simulink model "Y_Model_20_Loads"  (R2018b)
settings: Solver=VariableStepAuto  StartTime=0.0  StopTime=sim_t  RelTol=1e-3
values from neighbouring files (symbols this model uses):
  dt = 5e-5    (= 5e-05)    [Y_multi_sim_loads.m]
  L = ones(num_sims, num_loads) * L_max    [Y_multi_sim_loads.m]
  P = rand(num_sims, num_loads) * (P_max - P_min) + P_min    [Y_multi_sim_loads.m]
  R = ones(num_sims, num_loads) * R_max    [Y_multi_sim_loads.m]
libraries: powerlib x270, powerlib_meascontrol x56
(part 4 of 4)

== system Y_Model_20_Loads/PMU 7 ==
  "PMU (PLL-Based, Positive-Sequence)1" : powerlib_meascontrol/Measurements/PMU (PLL-Based, Positive-Sequence)  nominalFrequency=50  samplingRate=64  reportingFactor=64
      settings: SourceProductName=Simscape Electrical  SourceProductBaseCode=PS
  "PMU (PLL-Based, Positive-Sequence)2" : powerlib_meascontrol/Measurements/PMU (PLL-Based, Positive-Sequence)  nominalFrequency=50  samplingRate=64  reportingFactor=64
      settings: SourceProductName=Simscape Electrical  SourceProductBaseCode=PS
  Three-Phase V-I Measurement1 : powerlib/Measurements/Three-Phase V-I Measurement  VoltageMeasurement=phase-to-ground  SetLabelV=off  LabelV=Vabc  Vpu=off  VpuLL=off  CurrentMeasurement=no  SetLabelI=off  LabelI=Iabc  Ipu=off  Pbase=100e6  Vbase=500e3  OutputType=Complex  PhasorSimulation=off  PSBequivalent=0
      settings: SourceProductName=Simscape Electrical
  Three-Phase V-I Measurement25 : powerlib/Measurements/Three-Phase V-I Measurement  VoltageMeasurement=no  SetLabelV=off  LabelV=Vabc  Vpu=off  VpuLL=off  CurrentMeasurement=yes  SetLabelI=off  LabelI=Iabc  Ipu=off  Pbase=100e6  Vbase=500e3  OutputType=Complex  PhasorSimulation=off  PSBequivalent=0
      settings: SourceProductName=Simscape Electrical
  To Workspace1 : ToWorkspace  VariableName=i_mag7  SampleTime=-1
  To Workspace2 : ToWorkspace  VariableName=i_ang7  SampleTime=-1
  To Workspace3 : ToWorkspace  VariableName=v_mag7  SampleTime=-1
  To Workspace4 : ToWorkspace  VariableName=v_ang7  SampleTime=-1
  To Workspace5 : ToWorkspace  VariableName=v_freq7  SampleTime=-1
  To Workspace6 : ToWorkspace  VariableName=i_freq7  SampleTime=-1
  Connection Port : PMIOPort  Tag=PMCPort  Side=Left
  Connection Port1 : PMIOPort  Tag=PMCPort  Port=2  Side=Left
  Connection Port2 : PMIOPort  Tag=PMCPort  Port=3  Side=Left
  Connection Port3 : PMIOPort  Tag=PMCPort  Port=4  Side=Right
  Connection Port4 : PMIOPort  Tag=PMCPort  Port=5  Side=Right
  Connection Port5 : PMIOPort  Tag=PMCPort  Port=6  Side=Right
  wires:
  "PMU (PLL-Based, Positive-Sequence)1"/3 -> To Workspace5/1
  "PMU (PLL-Based, Positive-Sequence)1"/2 -> To Workspace4/1
  "PMU (PLL-Based, Positive-Sequence)1"/1 -> To Workspace3/1
  "PMU (PLL-Based, Positive-Sequence)2"/3 -> To Workspace6/1
  "PMU (PLL-Based, Positive-Sequence)2"/1 -> To Workspace1/1
  "PMU (PLL-Based, Positive-Sequence)2"/2 -> To Workspace2/1
  Three-Phase V-I Measurement25/1 -> "PMU (PLL-Based, Positive-Sequence)2"/1
  Three-Phase V-I Measurement1/1 -> "PMU (PLL-Based, Positive-Sequence)1"/1
  connections:
  Three-Phase V-I Measurement25/LConn1 -- Connection Port/RConn1 -- Three-Phase V-I Measurement1/LConn1
  Connection Port1/RConn1 -- Three-Phase V-I Measurement1/LConn2 -- Three-Phase V-I Measurement25/LConn2
  Connection Port2/RConn1 -- Three-Phase V-I Measurement25/LConn3 -- Three-Phase V-I Measurement1/LConn3
  Connection Port3/RConn1 -- Three-Phase V-I Measurement25/RConn1
  Three-Phase V-I Measurement25/RConn2 -- Connection Port4/RConn1
  Three-Phase V-I Measurement25/RConn3 -- Connection Port5/RConn1

== system Y_Model_20_Loads/PMU 8 ==
  "PMU (PLL-Based, Positive-Sequence)1" : powerlib_meascontrol/Measurements/PMU (PLL-Based, Positive-Sequence)  nominalFrequency=50  samplingRate=64  reportingFactor=64
      settings: SourceProductName=Simscape Electrical  SourceProductBaseCode=PS
  "PMU (PLL-Based, Positive-Sequence)2" : powerlib_meascontrol/Measurements/PMU (PLL-Based, Positive-Sequence)  nominalFrequency=50  samplingRate=64  reportingFactor=64
      settings: SourceProductName=Simscape Electrical  SourceProductBaseCode=PS
  Three-Phase V-I Measurement1 : powerlib/Measurements/Three-Phase V-I Measurement  VoltageMeasurement=phase-to-ground  SetLabelV=off  LabelV=Vabc  Vpu=off  VpuLL=off  CurrentMeasurement=no  SetLabelI=off  LabelI=Iabc  Ipu=off  Pbase=100e6  Vbase=500e3  OutputType=Complex  PhasorSimulation=off  PSBequivalent=0
      settings: SourceProductName=Simscape Electrical
  Three-Phase V-I Measurement25 : powerlib/Measurements/Three-Phase V-I Measurement  VoltageMeasurement=no  SetLabelV=off  LabelV=Vabc  Vpu=off  VpuLL=off  CurrentMeasurement=yes  SetLabelI=off  LabelI=Iabc  Ipu=off  Pbase=100e6  Vbase=500e3  OutputType=Complex  PhasorSimulation=off  PSBequivalent=0
      settings: SourceProductName=Simscape Electrical
  To Workspace1 : ToWorkspace  VariableName=i_mag8  SampleTime=-1
  To Workspace2 : ToWorkspace  VariableName=i_ang8  SampleTime=-1
  To Workspace3 : ToWorkspace  VariableName=v_mag8  SampleTime=-1
  To Workspace4 : ToWorkspace  VariableName=v_ang8  SampleTime=-1
  To Workspace5 : ToWorkspace  VariableName=v_freq8  SampleTime=-1
  To Workspace6 : ToWorkspace  VariableName=i_freq8  SampleTime=-1
  Connection Port : PMIOPort  Tag=PMCPort  Side=Left
  Connection Port1 : PMIOPort  Tag=PMCPort  Port=2  Side=Left
  Connection Port2 : PMIOPort  Tag=PMCPort  Port=3  Side=Left
  Connection Port3 : PMIOPort  Tag=PMCPort  Port=4  Side=Right
  Connection Port4 : PMIOPort  Tag=PMCPort  Port=5  Side=Right
  Connection Port5 : PMIOPort  Tag=PMCPort  Port=6  Side=Right
  wires:
  "PMU (PLL-Based, Positive-Sequence)1"/3 -> To Workspace5/1
  "PMU (PLL-Based, Positive-Sequence)1"/2 -> To Workspace4/1
  "PMU (PLL-Based, Positive-Sequence)1"/1 -> To Workspace3/1
  "PMU (PLL-Based, Positive-Sequence)2"/3 -> To Workspace6/1
  "PMU (PLL-Based, Positive-Sequence)2"/1 -> To Workspace1/1
  "PMU (PLL-Based, Positive-Sequence)2"/2 -> To Workspace2/1
  Three-Phase V-I Measurement25/1 -> "PMU (PLL-Based, Positive-Sequence)2"/1
  Three-Phase V-I Measurement1/1 -> "PMU (PLL-Based, Positive-Sequence)1"/1
  connections:
  Three-Phase V-I Measurement25/LConn1 -- Connection Port/RConn1 -- Three-Phase V-I Measurement1/LConn1
  Connection Port1/RConn1 -- Three-Phase V-I Measurement1/LConn2 -- Three-Phase V-I Measurement25/LConn2
  Connection Port2/RConn1 -- Three-Phase V-I Measurement25/LConn3 -- Three-Phase V-I Measurement1/LConn3
  Connection Port3/RConn1 -- Three-Phase V-I Measurement25/RConn1
  Three-Phase V-I Measurement25/RConn2 -- Connection Port4/RConn1
  Three-Phase V-I Measurement25/RConn3 -- Connection Port5/RConn1

== system Y_Model_20_Loads/PMU 9 ==
  "PMU (PLL-Based, Positive-Sequence)1" : powerlib_meascontrol/Measurements/PMU (PLL-Based, Positive-Sequence)  nominalFrequency=50  samplingRate=64  reportingFactor=64
      settings: SourceProductName=Simscape Electrical  SourceProductBaseCode=PS
  "PMU (PLL-Based, Positive-Sequence)2" : powerlib_meascontrol/Measurements/PMU (PLL-Based, Positive-Sequence)  nominalFrequency=50  samplingRate=64  reportingFactor=64
      settings: SourceProductName=Simscape Electrical  SourceProductBaseCode=PS
  Three-Phase V-I Measurement1 : powerlib/Measurements/Three-Phase V-I Measurement  VoltageMeasurement=phase-to-ground  SetLabelV=off  LabelV=Vabc  Vpu=off  VpuLL=off  CurrentMeasurement=no  SetLabelI=off  LabelI=Iabc  Ipu=off  Pbase=100e6  Vbase=500e3  OutputType=Complex  PhasorSimulation=off  PSBequivalent=0
      settings: SourceProductName=Simscape Electrical
  Three-Phase V-I Measurement25 : powerlib/Measurements/Three-Phase V-I Measurement  VoltageMeasurement=no  SetLabelV=off  LabelV=Vabc  Vpu=off  VpuLL=off  CurrentMeasurement=yes  SetLabelI=off  LabelI=Iabc  Ipu=off  Pbase=100e6  Vbase=500e3  OutputType=Complex  PhasorSimulation=off  PSBequivalent=0
      settings: SourceProductName=Simscape Electrical
  To Workspace1 : ToWorkspace  VariableName=i_mag9  SampleTime=-1
  To Workspace2 : ToWorkspace  VariableName=i_ang9  SampleTime=-1
  To Workspace3 : ToWorkspace  VariableName=v_mag9  SampleTime=-1
  To Workspace4 : ToWorkspace  VariableName=v_ang9  SampleTime=-1
  To Workspace5 : ToWorkspace  VariableName=v_freq9  SampleTime=-1
  To Workspace6 : ToWorkspace  VariableName=i_freq9  SampleTime=-1
  Connection Port : PMIOPort  Tag=PMCPort  Side=Left
  Connection Port1 : PMIOPort  Tag=PMCPort  Port=2  Side=Left
  Connection Port2 : PMIOPort  Tag=PMCPort  Port=3  Side=Left
  Connection Port3 : PMIOPort  Tag=PMCPort  Port=4  Side=Right
  Connection Port4 : PMIOPort  Tag=PMCPort  Port=5  Side=Right
  Connection Port5 : PMIOPort  Tag=PMCPort  Port=6  Side=Right
  wires:
  "PMU (PLL-Based, Positive-Sequence)1"/3 -> To Workspace5/1
  "PMU (PLL-Based, Positive-Sequence)1"/2 -> To Workspace4/1
  "PMU (PLL-Based, Positive-Sequence)1"/1 -> To Workspace3/1
  "PMU (PLL-Based, Positive-Sequence)2"/3 -> To Workspace6/1
  "PMU (PLL-Based, Positive-Sequence)2"/1 -> To Workspace1/1
  "PMU (PLL-Based, Positive-Sequence)2"/2 -> To Workspace2/1
  Three-Phase V-I Measurement25/1 -> "PMU (PLL-Based, Positive-Sequence)2"/1
  Three-Phase V-I Measurement1/1 -> "PMU (PLL-Based, Positive-Sequence)1"/1
  connections:
  Three-Phase V-I Measurement25/LConn1 -- Connection Port/RConn1 -- Three-Phase V-I Measurement1/LConn1
  Connection Port1/RConn1 -- Three-Phase V-I Measurement1/LConn2 -- Three-Phase V-I Measurement25/LConn2
  Connection Port2/RConn1 -- Three-Phase V-I Measurement25/LConn3 -- Three-Phase V-I Measurement1/LConn3
  Connection Port3/RConn1 -- Three-Phase V-I Measurement25/RConn1
  Three-Phase V-I Measurement25/RConn2 -- Connection Port4/RConn1
  Three-Phase V-I Measurement25/RConn3 -- Connection Port5/RConn1

== system Y_Model_20_Loads/SCADA 1 ==
  "PMU (PLL-Based, Positive-Sequence)1" : powerlib_meascontrol/Measurements/PMU (PLL-Based, Positive-Sequence)  nominalFrequency=50  samplingRate=64  reportingFactor=1280
      settings: SourceProductName=Simscape Electrical  SourceProductBaseCode=PS
  Three-Phase V-I Measurement1 : powerlib/Measurements/Three-Phase V-I Measurement  VoltageMeasurement=phase-to-ground  SetLabelV=off  LabelV=Vabc  Vpu=off  VpuLL=off  CurrentMeasurement=no  SetLabelI=off  LabelI=Iabc  Ipu=off  Pbase=100e6  Vbase=500e3  OutputType=Complex  PhasorSimulation=off  PSBequivalent=0
      settings: SourceProductName=Simscape Electrical
  To Workspace1 : ToWorkspace  VariableName=scada_ang1  SampleTime=-1
  To Workspace2 : ToWorkspace  VariableName=scada_mag1  SampleTime=-1
  To Workspace6 : ToWorkspace  VariableName=scada_freq1  SampleTime=-1
  Connection Port : PMIOPort  Tag=PMCPort  Side=Left
  Connection Port1 : PMIOPort  Tag=PMCPort  Port=2  Side=Left
  Connection Port2 : PMIOPort  Tag=PMCPort  Port=3  Side=Left
  Connection Port3 : PMIOPort  Tag=PMCPort  Port=4  Side=Right
  Connection Port4 : PMIOPort  Tag=PMCPort  Port=5  Side=Right
  Connection Port5 : PMIOPort  Tag=PMCPort  Port=6  Side=Right
  wires:
  Three-Phase V-I Measurement1/1 -> "PMU (PLL-Based, Positive-Sequence)1"/1
  "PMU (PLL-Based, Positive-Sequence)1"/1 -> To Workspace2/1
  "PMU (PLL-Based, Positive-Sequence)1"/2 -> To Workspace1/1
  "PMU (PLL-Based, Positive-Sequence)1"/3 -> To Workspace6/1
  connections:
  Connection Port/RConn1 -- Connection Port3/RConn1 -- Three-Phase V-I Measurement1/LConn1
  Connection Port1/RConn1 -- Connection Port4/RConn1 -- Three-Phase V-I Measurement1/LConn2
  Connection Port2/RConn1 -- Three-Phase V-I Measurement1/LConn3 -- Connection Port5/RConn1

== system Y_Model_20_Loads/SCADA 10 ==
  "PMU (PLL-Based, Positive-Sequence)1" : powerlib_meascontrol/Measurements/PMU (PLL-Based, Positive-Sequence)  nominalFrequency=50  samplingRate=64  reportingFactor=1280
      settings: SourceProductName=Simscape Electrical  SourceProductBaseCode=PS
  Three-Phase V-I Measurement1 : powerlib/Measurements/Three-Phase V-I Measurement  VoltageMeasurement=phase-to-ground  SetLabelV=off  LabelV=Vabc  Vpu=off  VpuLL=off  CurrentMeasurement=no  SetLabelI=off  LabelI=Iabc  Ipu=off  Pbase=100e6  Vbase=500e3  OutputType=Complex  PhasorSimulation=off  PSBequivalent=0
      settings: SourceProductName=Simscape Electrical
  To Workspace1 : ToWorkspace  VariableName=scada_ang10  SampleTime=-1
  To Workspace2 : ToWorkspace  VariableName=scada_mag10  SampleTime=-1
  To Workspace6 : ToWorkspace  VariableName=scada_freq10  SampleTime=-1
  Connection Port : PMIOPort  Tag=PMCPort  Side=Left
  Connection Port1 : PMIOPort  Tag=PMCPort  Port=2  Side=Left
  Connection Port2 : PMIOPort  Tag=PMCPort  Port=3  Side=Left
  Connection Port3 : PMIOPort  Tag=PMCPort  Port=4  Side=Right
  Connection Port4 : PMIOPort  Tag=PMCPort  Port=5  Side=Right
  Connection Port5 : PMIOPort  Tag=PMCPort  Port=6  Side=Right
  wires:
  Three-Phase V-I Measurement1/1 -> "PMU (PLL-Based, Positive-Sequence)1"/1
  "PMU (PLL-Based, Positive-Sequence)1"/1 -> To Workspace2/1
  "PMU (PLL-Based, Positive-Sequence)1"/2 -> To Workspace1/1
  "PMU (PLL-Based, Positive-Sequence)1"/3 -> To Workspace6/1
  connections:
  Connection Port/RConn1 -- Connection Port3/RConn1 -- Three-Phase V-I Measurement1/LConn1
  Connection Port1/RConn1 -- Connection Port4/RConn1 -- Three-Phase V-I Measurement1/LConn2
  Connection Port2/RConn1 -- Three-Phase V-I Measurement1/LConn3 -- Connection Port5/RConn1

== system Y_Model_20_Loads/SCADA 11 ==
  "PMU (PLL-Based, Positive-Sequence)1" : powerlib_meascontrol/Measurements/PMU (PLL-Based, Positive-Sequence)  nominalFrequency=50  samplingRate=64  reportingFactor=1280
      settings: SourceProductName=Simscape Electrical  SourceProductBaseCode=PS
  Three-Phase V-I Measurement1 : powerlib/Measurements/Three-Phase V-I Measurement  VoltageMeasurement=phase-to-ground  SetLabelV=off  LabelV=Vabc  Vpu=off  VpuLL=off  CurrentMeasurement=no  SetLabelI=off  LabelI=Iabc  Ipu=off  Pbase=100e6  Vbase=500e3  OutputType=Complex  PhasorSimulation=off  PSBequivalent=0
      settings: SourceProductName=Simscape Electrical
  To Workspace1 : ToWorkspace  VariableName=scada_ang11  SampleTime=-1
  To Workspace2 : ToWorkspace  VariableName=scada_mag11  SampleTime=-1
  To Workspace6 : ToWorkspace  VariableName=scada_freq11  SampleTime=-1
  Connection Port : PMIOPort  Tag=PMCPort  Side=Left
  Connection Port1 : PMIOPort  Tag=PMCPort  Port=2  Side=Left
  Connection Port2 : PMIOPort  Tag=PMCPort  Port=3  Side=Left
  Connection Port3 : PMIOPort  Tag=PMCPort  Port=4  Side=Right
  Connection Port4 : PMIOPort  Tag=PMCPort  Port=5  Side=Right
  Connection Port5 : PMIOPort  Tag=PMCPort  Port=6  Side=Right
  wires:
  Three-Phase V-I Measurement1/1 -> "PMU (PLL-Based, Positive-Sequence)1"/1
  "PMU (PLL-Based, Positive-Sequence)1"/1 -> To Workspace2/1
  "PMU (PLL-Based, Positive-Sequence)1"/2 -> To Workspace1/1
  "PMU (PLL-Based, Positive-Sequence)1"/3 -> To Workspace6/1
  connections:
  Connection Port/RConn1 -- Connection Port3/RConn1 -- Three-Phase V-I Measurement1/LConn1
  Connection Port1/RConn1 -- Connection Port4/RConn1 -- Three-Phase V-I Measurement1/LConn2
  Connection Port2/RConn1 -- Three-Phase V-I Measurement1/LConn3 -- Connection Port5/RConn1

== system Y_Model_20_Loads/SCADA 13 ==
  "PMU (PLL-Based, Positive-Sequence)1" : powerlib_meascontrol/Measurements/PMU (PLL-Based, Positive-Sequence)  nominalFrequency=50  samplingRate=64  reportingFactor=1280
      settings: SourceProductName=Simscape Electrical  SourceProductBaseCode=PS
  Three-Phase V-I Measurement1 : powerlib/Measurements/Three-Phase V-I Measurement  VoltageMeasurement=phase-to-ground  SetLabelV=off  LabelV=Vabc  Vpu=off  VpuLL=off  CurrentMeasurement=no  SetLabelI=off  LabelI=Iabc  Ipu=off  Pbase=100e6  Vbase=500e3  OutputType=Complex  PhasorSimulation=off  PSBequivalent=0
      settings: SourceProductName=Simscape Electrical
  To Workspace1 : ToWorkspace  VariableName=scada_ang13  SampleTime=-1
  To Workspace2 : ToWorkspace  VariableName=scada_mag13  SampleTime=-1
  To Workspace6 : ToWorkspace  VariableName=scada_freq13  SampleTime=-1
  Connection Port : PMIOPort  Tag=PMCPort  Side=Left
  Connection Port1 : PMIOPort  Tag=PMCPort  Port=2  Side=Left
  Connection Port2 : PMIOPort  Tag=PMCPort  Port=3  Side=Left
  Connection Port3 : PMIOPort  Tag=PMCPort  Port=4  Side=Right
  Connection Port4 : PMIOPort  Tag=PMCPort  Port=5  Side=Right
  Connection Port5 : PMIOPort  Tag=PMCPort  Port=6  Side=Right
  wires:
  Three-Phase V-I Measurement1/1 -> "PMU (PLL-Based, Positive-Sequence)1"/1
  "PMU (PLL-Based, Positive-Sequence)1"/1 -> To Workspace2/1
  "PMU (PLL-Based, Positive-Sequence)1"/2 -> To Workspace1/1
  "PMU (PLL-Based, Positive-Sequence)1"/3 -> To Workspace6/1
  connections:
  Connection Port/RConn1 -- Connection Port3/RConn1 -- Three-Phase V-I Measurement1/LConn1
  Connection Port1/RConn1 -- Connection Port4/RConn1 -- Three-Phase V-I Measurement1/LConn2
  Connection Port2/RConn1 -- Three-Phase V-I Measurement1/LConn3 -- Connection Port5/RConn1

== system Y_Model_20_Loads/SCADA 14 ==
  "PMU (PLL-Based, Positive-Sequence)1" : powerlib_meascontrol/Measurements/PMU (PLL-Based, Positive-Sequence)  nominalFrequency=50  samplingRate=64  reportingFactor=1280
      settings: SourceProductName=Simscape Electrical  SourceProductBaseCode=PS
  Three-Phase V-I Measurement1 : powerlib/Measurements/Three-Phase V-I Measurement  VoltageMeasurement=phase-to-ground  SetLabelV=off  LabelV=Vabc  Vpu=off  VpuLL=off  CurrentMeasurement=no  SetLabelI=off  LabelI=Iabc  Ipu=off  Pbase=100e6  Vbase=500e3  OutputType=Complex  PhasorSimulation=off  PSBequivalent=0
      settings: SourceProductName=Simscape Electrical
  To Workspace1 : ToWorkspace  VariableName=scada_ang14  SampleTime=-1
  To Workspace2 : ToWorkspace  VariableName=scada_mag14  SampleTime=-1
  To Workspace6 : ToWorkspace  VariableName=scada_freq14  SampleTime=-1
  Connection Port : PMIOPort  Tag=PMCPort  Side=Left
  Connection Port1 : PMIOPort  Tag=PMCPort  Port=2  Side=Left
  Connection Port2 : PMIOPort  Tag=PMCPort  Port=3  Side=Left
  Connection Port3 : PMIOPort  Tag=PMCPort  Port=4  Side=Right
  Connection Port4 : PMIOPort  Tag=PMCPort  Port=5  Side=Right
  Connection Port5 : PMIOPort  Tag=PMCPort  Port=6  Side=Right
  wires:
  Three-Phase V-I Measurement1/1 -> "PMU (PLL-Based, Positive-Sequence)1"/1
  "PMU (PLL-Based, Positive-Sequence)1"/1 -> To Workspace2/1
  "PMU (PLL-Based, Positive-Sequence)1"/2 -> To Workspace1/1
  "PMU (PLL-Based, Positive-Sequence)1"/3 -> To Workspace6/1
  connections:
  Connection Port/RConn1 -- Connection Port3/RConn1 -- Three-Phase V-I Measurement1/LConn1
  Connection Port1/RConn1 -- Connection Port4/RConn1 -- Three-Phase V-I Measurement1/LConn2
  Connection Port2/RConn1 -- Three-Phase V-I Measurement1/LConn3 -- Connection Port5/RConn1

== system Y_Model_20_Loads/SCADA 16 ==
  "PMU (PLL-Based, Positive-Sequence)1" : powerlib_meascontrol/Measurements/PMU (PLL-Based, Positive-Sequence)  nominalFrequency=50  samplingRate=64  reportingFactor=1280
      settings: SourceProductName=Simscape Electrical  SourceProductBaseCode=PS
  Three-Phase V-I Measurement1 : powerlib/Measurements/Three-Phase V-I Measurement  VoltageMeasurement=phase-to-ground  SetLabelV=off  LabelV=Vabc  Vpu=off  VpuLL=off  CurrentMeasurement=no  SetLabelI=off  LabelI=Iabc  Ipu=off  Pbase=100e6  Vbase=500e3  OutputType=Complex  PhasorSimulation=off  PSBequivalent=0
      settings: SourceProductName=Simscape Electrical
  To Workspace1 : ToWorkspace  VariableName=scada_ang16  SampleTime=-1
  To Workspace2 : ToWorkspace  VariableName=scada_mag16  SampleTime=-1
  To Workspace6 : ToWorkspace  VariableName=scada_freq16  SampleTime=-1
  Connection Port : PMIOPort  Tag=PMCPort  Side=Left
  Connection Port1 : PMIOPort  Tag=PMCPort  Port=2  Side=Left
  Connection Port2 : PMIOPort  Tag=PMCPort  Port=3  Side=Left
  Connection Port3 : PMIOPort  Tag=PMCPort  Port=4  Side=Right
  Connection Port4 : PMIOPort  Tag=PMCPort  Port=5  Side=Right
  Connection Port5 : PMIOPort  Tag=PMCPort  Port=6  Side=Right
  wires:
  Three-Phase V-I Measurement1/1 -> "PMU (PLL-Based, Positive-Sequence)1"/1
  "PMU (PLL-Based, Positive-Sequence)1"/1 -> To Workspace2/1
  "PMU (PLL-Based, Positive-Sequence)1"/2 -> To Workspace1/1
  "PMU (PLL-Based, Positive-Sequence)1"/3 -> To Workspace6/1
  connections:
  Connection Port/RConn1 -- Connection Port3/RConn1 -- Three-Phase V-I Measurement1/LConn1
  Connection Port1/RConn1 -- Connection Port4/RConn1 -- Three-Phase V-I Measurement1/LConn2
  Connection Port2/RConn1 -- Three-Phase V-I Measurement1/LConn3 -- Connection Port5/RConn1

== system Y_Model_20_Loads/SCADA 17 ==
  "PMU (PLL-Based, Positive-Sequence)1" : powerlib_meascontrol/Measurements/PMU (PLL-Based, Positive-Sequence)  nominalFrequency=50  samplingRate=64  reportingFactor=1280
      settings: SourceProductName=Simscape Electrical  SourceProductBaseCode=PS
  Three-Phase V-I Measurement1 : powerlib/Measurements/Three-Phase V-I Measurement  VoltageMeasurement=phase-to-ground  SetLabelV=off  LabelV=Vabc  Vpu=off  VpuLL=off  CurrentMeasurement=no  SetLabelI=off  LabelI=Iabc  Ipu=off  Pbase=100e6  Vbase=500e3  OutputType=Complex  PhasorSimulation=off  PSBequivalent=0
      settings: SourceProductName=Simscape Electrical
  To Workspace1 : ToWorkspace  VariableName=scada_ang17  SampleTime=-1
  To Workspace2 : ToWorkspace  VariableName=scada_mag17  SampleTime=-1
  To Workspace6 : ToWorkspace  VariableName=scada_freq17  SampleTime=-1
  Connection Port : PMIOPort  Tag=PMCPort  Side=Left
  Connection Port1 : PMIOPort  Tag=PMCPort  Port=2  Side=Left
  Connection Port2 : PMIOPort  Tag=PMCPort  Port=3  Side=Left
  Connection Port3 : PMIOPort  Tag=PMCPort  Port=4  Side=Right
  Connection Port4 : PMIOPort  Tag=PMCPort  Port=5  Side=Right
  Connection Port5 : PMIOPort  Tag=PMCPort  Port=6  Side=Right
  wires:
  Three-Phase V-I Measurement1/1 -> "PMU (PLL-Based, Positive-Sequence)1"/1
  "PMU (PLL-Based, Positive-Sequence)1"/1 -> To Workspace2/1
  "PMU (PLL-Based, Positive-Sequence)1"/2 -> To Workspace1/1
  "PMU (PLL-Based, Positive-Sequence)1"/3 -> To Workspace6/1
  connections:
  Connection Port/RConn1 -- Connection Port3/RConn1 -- Three-Phase V-I Measurement1/LConn1
  Connection Port1/RConn1 -- Connection Port4/RConn1 -- Three-Phase V-I Measurement1/LConn2
  Connection Port2/RConn1 -- Three-Phase V-I Measurement1/LConn3 -- Connection Port5/RConn1

== system Y_Model_20_Loads/SCADA 19 ==
  "PMU (PLL-Based, Positive-Sequence)1" : powerlib_meascontrol/Measurements/PMU (PLL-Based, Positive-Sequence)  nominalFrequency=50  samplingRate=64  reportingFactor=1280
      settings: SourceProductName=Simscape Electrical  SourceProductBaseCode=PS
  Three-Phase V-I Measurement1 : powerlib/Measurements/Three-Phase V-I Measurement  VoltageMeasurement=phase-to-ground  SetLabelV=off  LabelV=Vabc  Vpu=off  VpuLL=off  CurrentMeasurement=no  SetLabelI=off  LabelI=Iabc  Ipu=off  Pbase=100e6  Vbase=500e3  OutputType=Complex  PhasorSimulation=off  PSBequivalent=0
      settings: SourceProductName=Simscape Electrical
  To Workspace1 : ToWorkspace  VariableName=scada_ang19  SampleTime=-1
  To Workspace2 : ToWorkspace  VariableName=scada_mag19  SampleTime=-1
  To Workspace6 : ToWorkspace  VariableName=scada_freq19  SampleTime=-1
  Connection Port : PMIOPort  Tag=PMCPort  Side=Left
  Connection Port1 : PMIOPort  Tag=PMCPort  Port=2  Side=Left
  Connection Port2 : PMIOPort  Tag=PMCPort  Port=3  Side=Left
  Connection Port3 : PMIOPort  Tag=PMCPort  Port=4  Side=Right
  Connection Port4 : PMIOPort  Tag=PMCPort  Port=5  Side=Right
  Connection Port5 : PMIOPort  Tag=PMCPort  Port=6  Side=Right
  wires:
  Three-Phase V-I Measurement1/1 -> "PMU (PLL-Based, Positive-Sequence)1"/1
  "PMU (PLL-Based, Positive-Sequence)1"/1 -> To Workspace2/1
  "PMU (PLL-Based, Positive-Sequence)1"/2 -> To Workspace1/1
  "PMU (PLL-Based, Positive-Sequence)1"/3 -> To Workspace6/1
  connections:
  Connection Port/RConn1 -- Connection Port3/RConn1 -- Three-Phase V-I Measurement1/LConn1
  Connection Port1/RConn1 -- Connection Port4/RConn1 -- Three-Phase V-I Measurement1/LConn2
  Connection Port2/RConn1 -- Three-Phase V-I Measurement1/LConn3 -- Connection Port5/RConn1

== system Y_Model_20_Loads/SCADA 2 ==
  "PMU (PLL-Based, Positive-Sequence)1" : powerlib_meascontrol/Measurements/PMU (PLL-Based, Positive-Sequence)  nominalFrequency=50  samplingRate=64  reportingFactor=1280
      settings: SourceProductName=Simscape Electrical  SourceProductBaseCode=PS
  Three-Phase V-I Measurement1 : powerlib/Measurements/Three-Phase V-I Measurement  VoltageMeasurement=phase-to-ground  SetLabelV=off  LabelV=Vabc  Vpu=off  VpuLL=off  CurrentMeasurement=no  SetLabelI=off  LabelI=Iabc  Ipu=off  Pbase=100e6  Vbase=500e3  OutputType=Complex  PhasorSimulation=off  PSBequivalent=0
      settings: SourceProductName=Simscape Electrical
  To Workspace1 : ToWorkspace  VariableName=scada_ang2  SampleTime=-1
  To Workspace2 : ToWorkspace  VariableName=scada_mag2  SampleTime=-1
  To Workspace6 : ToWorkspace  VariableName=scada_freq2  SampleTime=-1
  Connection Port : PMIOPort  Tag=PMCPort  Side=Left
  Connection Port1 : PMIOPort  Tag=PMCPort  Port=2  Side=Left
  Connection Port2 : PMIOPort  Tag=PMCPort  Port=3  Side=Left
  Connection Port3 : PMIOPort  Tag=PMCPort  Port=4  Side=Right
  Connection Port4 : PMIOPort  Tag=PMCPort  Port=5  Side=Right
  Connection Port5 : PMIOPort  Tag=PMCPort  Port=6  Side=Right
  wires:
  Three-Phase V-I Measurement1/1 -> "PMU (PLL-Based, Positive-Sequence)1"/1
  "PMU (PLL-Based, Positive-Sequence)1"/1 -> To Workspace2/1
  "PMU (PLL-Based, Positive-Sequence)1"/2 -> To Workspace1/1
  "PMU (PLL-Based, Positive-Sequence)1"/3 -> To Workspace6/1
  connections:
  Connection Port/RConn1 -- Connection Port3/RConn1 -- Three-Phase V-I Measurement1/LConn1
  Connection Port1/RConn1 -- Connection Port4/RConn1 -- Three-Phase V-I Measurement1/LConn2
  Connection Port2/RConn1 -- Three-Phase V-I Measurement1/LConn3 -- Connection Port5/RConn1

== system Y_Model_20_Loads/SCADA 20 ==
  "PMU (PLL-Based, Positive-Sequence)1" : powerlib_meascontrol/Measurements/PMU (PLL-Based, Positive-Sequence)  nominalFrequency=50  samplingRate=64  reportingFactor=1280
      settings: SourceProductName=Simscape Electrical  SourceProductBaseCode=PS
  Three-Phase V-I Measurement1 : powerlib/Measurements/Three-Phase V-I Measurement  VoltageMeasurement=phase-to-ground  SetLabelV=off  LabelV=Vabc  Vpu=off  VpuLL=off  CurrentMeasurement=no  SetLabelI=off  LabelI=Iabc  Ipu=off  Pbase=100e6  Vbase=500e3  OutputType=Complex  PhasorSimulation=off  PSBequivalent=0
      settings: SourceProductName=Simscape Electrical
  To Workspace1 : ToWorkspace  VariableName=scada_ang20  SampleTime=-1
  To Workspace2 : ToWorkspace  VariableName=scada_mag20  SampleTime=-1
  To Workspace6 : ToWorkspace  VariableName=scada_freq20  SampleTime=-1
  Connection Port : PMIOPort  Tag=PMCPort  Side=Left
  Connection Port1 : PMIOPort  Tag=PMCPort  Port=2  Side=Left
  Connection Port2 : PMIOPort  Tag=PMCPort  Port=3  Side=Left
  Connection Port3 : PMIOPort  Tag=PMCPort  Port=4  Side=Right
  Connection Port4 : PMIOPort  Tag=PMCPort  Port=5  Side=Right
  Connection Port5 : PMIOPort  Tag=PMCPort  Port=6  Side=Right
  wires:
  Three-Phase V-I Measurement1/1 -> "PMU (PLL-Based, Positive-Sequence)1"/1
  "PMU (PLL-Based, Positive-Sequence)1"/1 -> To Workspace2/1
  "PMU (PLL-Based, Positive-Sequence)1"/2 -> To Workspace1/1
  "PMU (PLL-Based, Positive-Sequence)1"/3 -> To Workspace6/1
  connections:
  Connection Port/RConn1 -- Connection Port3/RConn1 -- Three-Phase V-I Measurement1/LConn1
  Connection Port1/RConn1 -- Connection Port4/RConn1 -- Three-Phase V-I Measurement1/LConn2
  Connection Port2/RConn1 -- Three-Phase V-I Measurement1/LConn3 -- Connection Port5/RConn1

== system Y_Model_20_Loads/SCADA 4 ==
  "PMU (PLL-Based, Positive-Sequence)1" : powerlib_meascontrol/Measurements/PMU (PLL-Based, Positive-Sequence)  nominalFrequency=50  samplingRate=64  reportingFactor=1280
      settings: SourceProductName=Simscape Electrical  SourceProductBaseCode=PS
  Three-Phase V-I Measurement1 : powerlib/Measurements/Three-Phase V-I Measurement  VoltageMeasurement=phase-to-ground  SetLabelV=off  LabelV=Vabc  Vpu=off  VpuLL=off  CurrentMeasurement=no  SetLabelI=off  LabelI=Iabc  Ipu=off  Pbase=100e6  Vbase=500e3  OutputType=Complex  PhasorSimulation=off  PSBequivalent=0
      settings: SourceProductName=Simscape Electrical
  To Workspace1 : ToWorkspace  VariableName=scada_ang4  SampleTime=-1
  To Workspace2 : ToWorkspace  VariableName=scada_mag4  SampleTime=-1
  To Workspace6 : ToWorkspace  VariableName=scada_freq4  SampleTime=-1
  Connection Port : PMIOPort  Tag=PMCPort  Side=Left
  Connection Port1 : PMIOPort  Tag=PMCPort  Port=2  Side=Left
  Connection Port2 : PMIOPort  Tag=PMCPort  Port=3  Side=Left
  Connection Port3 : PMIOPort  Tag=PMCPort  Port=4  Side=Right
  Connection Port4 : PMIOPort  Tag=PMCPort  Port=5  Side=Right
  Connection Port5 : PMIOPort  Tag=PMCPort  Port=6  Side=Right
  wires:
  Three-Phase V-I Measurement1/1 -> "PMU (PLL-Based, Positive-Sequence)1"/1
  "PMU (PLL-Based, Positive-Sequence)1"/1 -> To Workspace2/1
  "PMU (PLL-Based, Positive-Sequence)1"/2 -> To Workspace1/1
  "PMU (PLL-Based, Positive-Sequence)1"/3 -> To Workspace6/1
  connections:
  Connection Port/RConn1 -- Connection Port3/RConn1 -- Three-Phase V-I Measurement1/LConn1
  Connection Port1/RConn1 -- Connection Port4/RConn1 -- Three-Phase V-I Measurement1/LConn2
  Connection Port2/RConn1 -- Three-Phase V-I Measurement1/LConn3 -- Connection Port5/RConn1

== system Y_Model_20_Loads/SCADA 5 ==
  "PMU (PLL-Based, Positive-Sequence)1" : powerlib_meascontrol/Measurements/PMU (PLL-Based, Positive-Sequence)  nominalFrequency=50  samplingRate=64  reportingFactor=1280
      settings: SourceProductName=Simscape Electrical  SourceProductBaseCode=PS
  Three-Phase V-I Measurement1 : powerlib/Measurements/Three-Phase V-I Measurement  VoltageMeasurement=phase-to-ground  SetLabelV=off  LabelV=Vabc  Vpu=off  VpuLL=off  CurrentMeasurement=no  SetLabelI=off  LabelI=Iabc  Ipu=off  Pbase=100e6  Vbase=500e3  OutputType=Complex  PhasorSimulation=off  PSBequivalent=0
      settings: SourceProductName=Simscape Electrical
  To Workspace1 : ToWorkspace  VariableName=scada_ang5  SampleTime=-1
  To Workspace2 : ToWorkspace  VariableName=scada_mag5  SampleTime=-1
  To Workspace6 : ToWorkspace  VariableName=scada_freq5  SampleTime=-1
  Connection Port : PMIOPort  Tag=PMCPort  Side=Left
  Connection Port1 : PMIOPort  Tag=PMCPort  Port=2  Side=Left
  Connection Port2 : PMIOPort  Tag=PMCPort  Port=3  Side=Left
  Connection Port3 : PMIOPort  Tag=PMCPort  Port=4  Side=Right
  Connection Port4 : PMIOPort  Tag=PMCPort  Port=5  Side=Right
  Connection Port5 : PMIOPort  Tag=PMCPort  Port=6  Side=Right
  wires:
  Three-Phase V-I Measurement1/1 -> "PMU (PLL-Based, Positive-Sequence)1"/1
  "PMU (PLL-Based, Positive-Sequence)1"/1 -> To Workspace2/1
  "PMU (PLL-Based, Positive-Sequence)1"/2 -> To Workspace1/1
  "PMU (PLL-Based, Positive-Sequence)1"/3 -> To Workspace6/1
  connections:
  Connection Port/RConn1 -- Connection Port3/RConn1 -- Three-Phase V-I Measurement1/LConn1
  Connection Port1/RConn1 -- Connection Port4/RConn1 -- Three-Phase V-I Measurement1/LConn2
  Connection Port2/RConn1 -- Three-Phase V-I Measurement1/LConn3 -- Connection Port5/RConn1

== system Y_Model_20_Loads/SCADA 7 ==
  "PMU (PLL-Based, Positive-Sequence)1" : powerlib_meascontrol/Measurements/PMU (PLL-Based, Positive-Sequence)  nominalFrequency=50  samplingRate=64  reportingFactor=1280
      settings: SourceProductName=Simscape Electrical  SourceProductBaseCode=PS
  Three-Phase V-I Measurement1 : powerlib/Measurements/Three-Phase V-I Measurement  VoltageMeasurement=phase-to-ground  SetLabelV=off  LabelV=Vabc  Vpu=off  VpuLL=off  CurrentMeasurement=no  SetLabelI=off  LabelI=Iabc  Ipu=off  Pbase=100e6  Vbase=500e3  OutputType=Complex  PhasorSimulation=off  PSBequivalent=0
      settings: SourceProductName=Simscape Electrical
  To Workspace1 : ToWorkspace  VariableName=scada_ang7  SampleTime=-1
  To Workspace2 : ToWorkspace  VariableName=scada_mag7  SampleTime=-1
  To Workspace6 : ToWorkspace  VariableName=scada_freq7  SampleTime=-1
  Connection Port : PMIOPort  Tag=PMCPort  Side=Left
  Connection Port1 : PMIOPort  Tag=PMCPort  Port=2  Side=Left
  Connection Port2 : PMIOPort  Tag=PMCPort  Port=3  Side=Left
  Connection Port3 : PMIOPort  Tag=PMCPort  Port=4  Side=Right
  Connection Port4 : PMIOPort  Tag=PMCPort  Port=5  Side=Right
  Connection Port5 : PMIOPort  Tag=PMCPort  Port=6  Side=Right
  wires:
  Three-Phase V-I Measurement1/1 -> "PMU (PLL-Based, Positive-Sequence)1"/1
  "PMU (PLL-Based, Positive-Sequence)1"/1 -> To Workspace2/1
  "PMU (PLL-Based, Positive-Sequence)1"/2 -> To Workspace1/1
  "PMU (PLL-Based, Positive-Sequence)1"/3 -> To Workspace6/1
  connections:
  Connection Port/RConn1 -- Connection Port3/RConn1 -- Three-Phase V-I Measurement1/LConn1
  Connection Port1/RConn1 -- Connection Port4/RConn1 -- Three-Phase V-I Measurement1/LConn2
  Connection Port2/RConn1 -- Three-Phase V-I Measurement1/LConn3 -- Connection Port5/RConn1

== system Y_Model_20_Loads/SCADA 8 ==
  "PMU (PLL-Based, Positive-Sequence)1" : powerlib_meascontrol/Measurements/PMU (PLL-Based, Positive-Sequence)  nominalFrequency=50  samplingRate=64  reportingFactor=1280
      settings: SourceProductName=Simscape Electrical  SourceProductBaseCode=PS
  Three-Phase V-I Measurement1 : powerlib/Measurements/Three-Phase V-I Measurement  VoltageMeasurement=phase-to-ground  SetLabelV=off  LabelV=Vabc  Vpu=off  VpuLL=off  CurrentMeasurement=no  SetLabelI=off  LabelI=Iabc  Ipu=off  Pbase=100e6  Vbase=500e3  OutputType=Complex  PhasorSimulation=off  PSBequivalent=0
      settings: SourceProductName=Simscape Electrical
  To Workspace1 : ToWorkspace  VariableName=scada_ang8  SampleTime=-1
  To Workspace2 : ToWorkspace  VariableName=scada_mag8  SampleTime=-1
  To Workspace6 : ToWorkspace  VariableName=scada_freq8  SampleTime=-1
  Connection Port : PMIOPort  Tag=PMCPort  Side=Left
  Connection Port1 : PMIOPort  Tag=PMCPort  Port=2  Side=Left
  Connection Port2 : PMIOPort  Tag=PMCPort  Port=3  Side=Left
  Connection Port3 : PMIOPort  Tag=PMCPort  Port=4  Side=Right
  Connection Port4 : PMIOPort  Tag=PMCPort  Port=5  Side=Right
  Connection Port5 : PMIOPort  Tag=PMCPort  Port=6  Side=Right
  wires:
  Three-Phase V-I Measurement1/1 -> "PMU (PLL-Based, Positive-Sequence)1"/1
  "PMU (PLL-Based, Positive-Sequence)1"/1 -> To Workspace2/1
  "PMU (PLL-Based, Positive-Sequence)1"/2 -> To Workspace1/1
  "PMU (PLL-Based, Positive-Sequence)1"/3 -> To Workspace6/1
  connections:
  Connection Port/RConn1 -- Connection Port3/RConn1 -- Three-Phase V-I Measurement1/LConn1
  Connection Port1/RConn1 -- Connection Port4/RConn1 -- Three-Phase V-I Measurement1/LConn2
  Connection Port2/RConn1 -- Three-Phase V-I Measurement1/LConn3 -- Connection Port5/RConn1
